simulink model "P3"  (R2023a)
settings: Solver=VariableStepAuto  StartTime=0.0  StopTime=10.0  RelTol=1e-3
model workspace (MAT data in the model file):
  b1 = 1000
  k1 = 16182
  k2 = 19000
  m1 = 290
  m2 = 59
  z = 1
  z1 = Simulink.Parameter
  z1.DataType = 'auto'
  z1.Complexity = 'real'
  z1.Dimensions = [0 0]

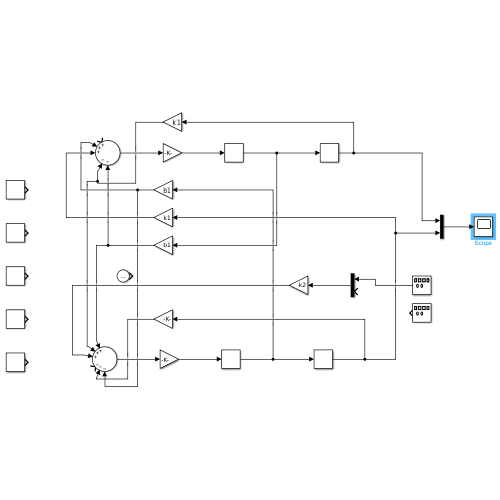
[thumbnail: Simulink's stored preview of the top-level diagram]
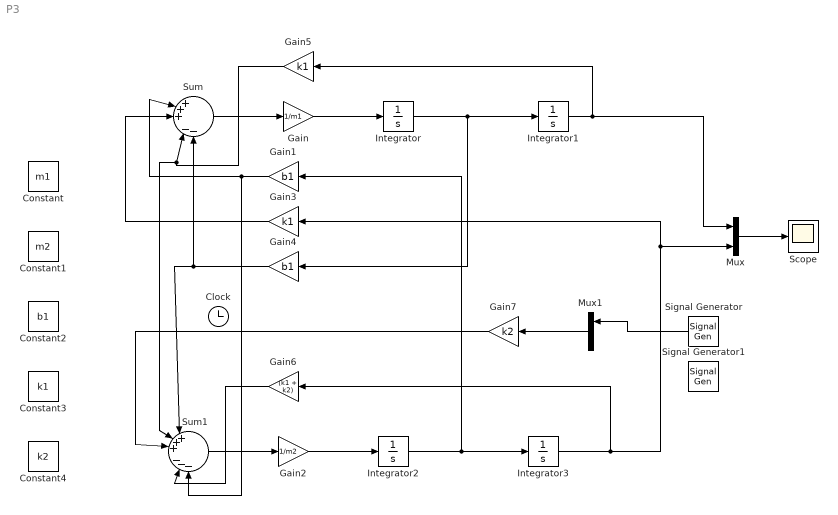
== system P3 ==
  Clock : Clock
  Constant : Constant  Value=m1
  Constant1 : Constant  Value=m2
  Constant2 : Constant  Value=b1
  Constant3 : Constant  Value=k1
  Constant4 : Constant  Value=k2
  Gain : Gain  Gain=1/m1
  Gain1 : Gain  Gain=b1
  Gain2 : Gain  Gain=1/m2
  Gain3 : Gain  Gain=k1
  Gain4 : Gain  Gain=b1
  Gain5 : Gain  Gain=k1
  Gain6 : Gain  Gain=(k1 + k2)
  Gain7 : Gain  Gain=k2
  Integrator{,1..3} (4 alike) : Integrator
  Mux : Mux  Inputs=2
  Mux1 : Mux  Inputs=2
  Scope : Scope
  Signal Generator : SignalGenerator  Amplitude=0.05  Frequency=0.5*3.1416  Units=rad/sec
  Signal Generator1 : SignalGenerator  Amplitude=0.05  Frequency=20*3.1416  Units=rad/sec
  Sum : Sum  Inputs=|+++|--
  Sum1 : Sum  Inputs=|+++|---
  wires:
  Integrator/1 -> Gain4/1, Integrator1/1
  Gain/1 -> Integrator/1
  Sum/1 -> Gain/1
  Gain2/1 -> Integrator2/1
  Sum1/1 -> Gain2/1
  Integrator2/1 -> Gain1/1, Integrator3/1
  Gain1/1 -> Sum1/6, Sum/2
  Integrator3/1 -> Gain6/1, Mux/2, Gain3/1
  Gain3/1 -> Sum/3
  Gain4/1 -> Sum1/1, Sum/5
  Integrator1/1 -> Mux/1, Gain5/1
  Gain5/1 -> Sum1/2, Sum/4
  Gain6/1 -> Sum1/5
  Mux/1 -> Scope/1
  Gain7/1 -> Sum1/3
  Mux1/1 -> Gain7/1
  Signal Generator/1 -> Mux1/1
